simulink model "dPTPUDPNode1_tm"  (R2018b)
settings: Solver=FixedStepDiscrete  StartTime=0.0  StopTime=inf  FixedStep=0.01  RelTol=1e-3  EnableMultiTasking=on
undefined symbols (not defined in the file): ipaddr, PTP
libraries: xpcutilitieslib x6, xpcrtudplib x6, ptplib x3
settings Model: SimulationMode=external  Creator=The MathWorks, Inc.  LastModifiedBy=MAE-NCSUCORE
settings SolverCC: ConcurrentTasks=on  AutoInsertRateTranBlk=on  DecoupledContinuousIntegration=on  MinimalZcImpactIntegration=on
settings DataIOCC: SaveFormat=StructureWithTime
settings OptimizationCC: BlockReduction=off  OptimizeBlockIOStorage=off  BufferReuse=off  GlobalBufferReuse=off  ExpressionFolding=off  LocalBlockOutputs=off  OptimizeDataStoreBuffers=off  BusAssignmentInplaceUpdate=off
settings DebuggingCC: LibraryContextMissingDiagnostic=none
settings HardwareCC: ProdBitPerPointer=32  ProdBitPerSizeT=32  ProdBitPerPtrDiffT=32  ProdLargestAtomicFloat=None  ProdWordSize=32  ProdLongLongMode=on  ProdHWDeviceType=Generic->32-bit x86 compatible
settings SFSimCC: SimUseLocalCustomCode=off
settings RTWCC: SystemTargetFile=slrt.tlc  TemplateMakefile=slrt_default_tmf  Description=Simulink Real-Time  RTWVerbose=off  RTWUseLocalCustomCode=off  CodeExecutionProfiling=on  RTWCompilerOptimization=on
settings SimulinkRealTimeCC: SupportVariableSizeSignals=on  PreserveStateflowLocalDataDimensions=off  RL32LogTETModifier=off  RL32ObjectName=tg1  xPCisDefaultEnv=off  xPCTargetPCEnvName=Machine2  xPCConcurrentTasks=on

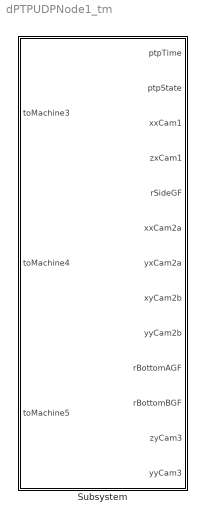
== system dPTPUDPNode1_tm ==
  Subsystem : Subsystem  TreatAsAtomicUnit=on  mask{sample_time=0.01, announce_interval=1, sync_interval=0.05}
      mask prompts: sample_time "Sample time (-1 for inherited)"; announce_interval "Announce interval (second):"; sync_interval "Sync interval (second):"
      mask TypeOptions sample_time: IEEE 1588 Read State/sample_time | IEEE 1588 Read Time/sample_time | IEEE 1588 Real-Time UDP/sample_time | UDP Receive Machine 3/sampleTime | UDP Receive Machine 4/sampleTime | UDP Receive Machine 5/sampleTime | UDP Send Machine 3/sampleTime | UDP Send Machine 4/sampleTime | UDP Send Machine 5/sampleTime
      mask TypeOptions announce_interval: IEEE 1588 Real-Time UDP/announce_interval
      mask TypeOptions sync_interval: IEEE 1588 Real-Time UDP/sync_interval

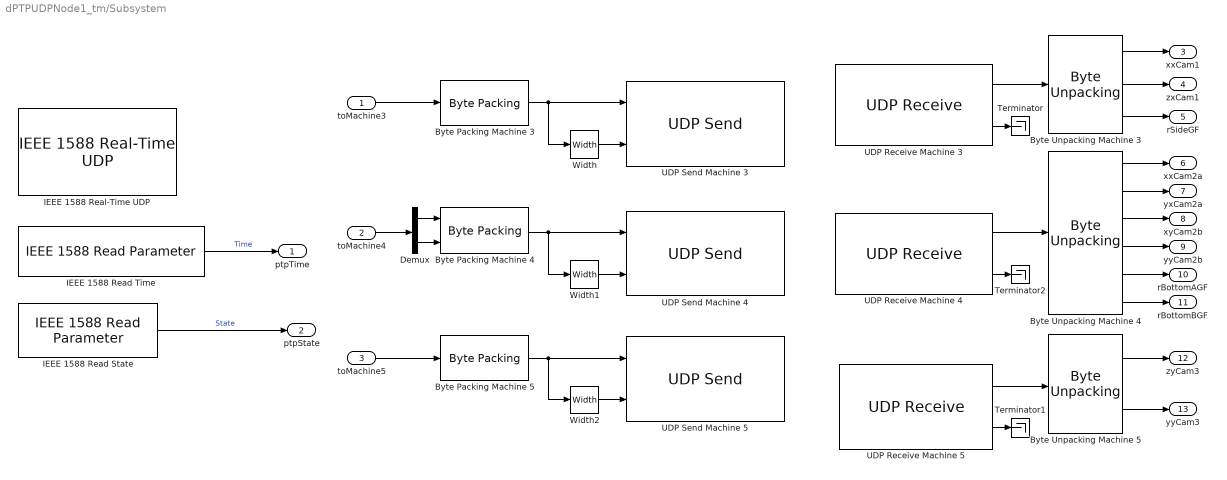
== system dPTPUDPNode1_tm/Subsystem ==
  toMachine3 : Inport
  toMachine4 : Inport  Port=2
  toMachine5 : Inport  Port=3
  Byte Packing Machine 3 : xpcutilitieslib/Byte Packing   MaskPackedDataType=uint8  MaskUnpackedDataTypes={['uint8']}  MaskAlignment=1
  Byte Packing Machine 4 : xpcutilitieslib/Byte Packing   MaskPackedDataType=uint8  MaskUnpackedDataTypes={['uint8'],['uint8']}  MaskAlignment=1
  Byte Packing Machine 5 : xpcutilitieslib/Byte Packing   MaskPackedDataType=uint8  MaskUnpackedDataTypes={['uint8']}  MaskAlignment=1
  "Byte Unpacking Machine 3 " : xpcutilitieslib/Byte Unpacking   MaskUnpackedDataTypes={'double','double',['uint8']}  MaskUnpackedDataSizes={[1],[1],[3]}  MaskAlignment=1
      settings: SourceProductName=Simulink Real-Time  SourceProductBaseCode=XP
  Byte Unpacking Machine 4 : xpcutilitieslib/Byte Unpacking   MaskUnpackedDataTypes={'double','double','double','double',['uint8'],['uint8']}  MaskUnpackedDataSizes={[1],[1],[1],[1],[3],[3]}  MaskAlignment=1
      settings: SourceProductName=Simulink Real-Time  SourceProductBaseCode=XP
  Byte Unpacking Machine 5 : xpcutilitieslib/Byte Unpacking   MaskUnpackedDataTypes={'double','double'}  MaskUnpackedDataSizes={[1],[1]}  MaskAlignment=1
      settings: SourceProductName=Simulink Real-Time  SourceProductBaseCode=XP
  Demux : Demux  Outputs=2
  IEEE 1588 Read State : ptplib/IEEE 1588 Read Parameter  Priority=1  ID=1  param=Protocol state  sample_time=sample_time  enable_read_precision=off
      settings: SourceProductName=Simulink Real-Time  SourceProductBaseCode=XP
  IEEE 1588 Read Time : ptplib/IEEE 1588 Read Parameter  Priority=1  ID=1  param=PTP time (time-of-day)  sample_time=sample_time  enable_read_precision=off
      settings: SourceProductName=Simulink Real-Time  SourceProductBaseCode=XP
  IEEE 1588 Real-Time UDP : ptplib/IEEE 1588 Real-Time UDP  Priority=0  ID=1  PciBus=2  PciSlot=0  PciFunction=0  time_inc=4000000  sample_time=sample_time  IpSource=Specify  IpAddress=30.30.30.30  SubnetMask=255.255.255.0  Gateway=0.0.0.0  Receive1=0.0.0.0  dest_ip_select=Specify  custom_dest_ip_addr=255.255.255.255  MulticastList=[ipaddr('224.0.1.129'), ipaddr('224.0.0.107')]  Multicast={macaddr('01:00:5E:00:01:81'), macaddr('01:00:5E:00:00:6B')}  time_source=Ethernet board  timescale=PTP (1970-01-01)  epoch=[1970 01 01 00]  delay_measure=Request-response  slave_only=off  enable_advanced_config=on  domain_num=0  utc_offset=35  priority1=1  clock_class=248  clock_accuracy=hex2dec('FE')  priority2=1  announce_interval=announce_interval  sync_interval=sync_interval  min_pdelay_req_interval=0.1  announce_receipt_timeout=3
      settings: SourceProductName=Simulink Real-Time  SourceProductBaseCode=XP
  Terminator : Terminator
  Terminator1 : Terminator
  Terminator2 : Terminator
  UDP Receive Machine 3 : xpcrtudplib/UDP Receive  ipAddressVal=30.30.30.30  localPort=8001  rcvWidth=8  rcvFmAny=off  fmAddress=30.30.30.1  rcvMulticast=off  multicastAddress={30.30.30.1, 30.30.30.2, 30.30.30.3}  maxUDPQueue=8  sampleTime=sample_time
      settings: SourceProductName=Simulink Real-Time
  UDP Receive Machine 4 : xpcrtudplib/UDP Receive  ipAddressVal=30.30.30.30  localPort=8002  rcvWidth=8  rcvFmAny=off  fmAddress=30.30.30.2  rcvMulticast=off  multicastAddress={30.30.30.1, 30.30.30.2, 30.30.30.3}  maxUDPQueue=8  sampleTime=sample_time
      settings: SourceProductName=Simulink Real-Time
  UDP Receive Machine 5 : xpcrtudplib/UDP Receive  ipAddressVal=30.30.30.30  localPort=8003  rcvWidth=8  rcvFmAny=off  fmAddress=30.30.30.3  rcvMulticast=off  multicastAddress={30.30.30.1, 30.30.30.2, 30.30.30.3}  maxUDPQueue=8  sampleTime=sample_time
      settings: SourceProductName=Simulink Real-Time
  UDP Send Machine 3 : xpcrtudplib/UDP Send  ipAddressVal=30.30.30.30  localPort=8001  toAddress=30.30.30.1  toPort=8000  sampleTime=sample_time
      settings: SourceProductName=Simulink Real-Time  SourceProductBaseCode=XP
  UDP Send Machine 4 : xpcrtudplib/UDP Send  ipAddressVal=30.30.30.30  localPort=8002  toAddress=30.30.30.2  toPort=8000  sampleTime=sample_time
      settings: SourceProductName=Simulink Real-Time  SourceProductBaseCode=XP
  UDP Send Machine 5 : xpcrtudplib/UDP Send  ipAddressVal=30.30.30.30  localPort=8003  toAddress=30.30.30.3  toPort=8000  sampleTime=sample_time
      settings: SourceProductName=Simulink Real-Time  SourceProductBaseCode=XP
  Width : Width
  Width1 : Width
  Width2 : Width
  ptpTime : Outport
  ptpState : Outport  Port=2
  xxCam1 : Outport  Port=3
  zxCam1 : Outport  Port=4
  rSideGF : Outport  Port=5
  xxCam2a : Outport  Port=6
  yxCam2a : Outport  Port=7
  xyCam2b : Outport  Port=8
  yyCam2b : Outport  Port=9
  rBottomAGF : Outport  Port=10
  rBottomBGF : Outport  Port=11
  zyCam3 : Outport  Port=12
  yyCam3 : Outport  Port=13
  wires:
  Byte Unpacking Machine 4/1 -> xxCam2a/1
  Byte Unpacking Machine 4/6 -> rBottomBGF/1
  Byte Unpacking Machine 4/3 -> xyCam2b/1
  UDP Receive Machine 5/1 -> Byte Unpacking Machine 5/1
  "Byte Unpacking Machine 3 "/3 -> rSideGF/1
  toMachine3/1 -> Byte Packing Machine 3/1
  IEEE 1588 Read State/1 -> ptpState/1  "State"
  "Byte Unpacking Machine 3 "/2 -> zxCam1/1
  toMachine5/1 -> Byte Packing Machine 5/1
  toMachine4/1 -> Demux/1
  Demux/2 -> Byte Packing Machine 4/2
  Byte Unpacking Machine 5/1 -> zyCam3/1
  UDP Receive Machine 4/2 -> Terminator2/1
  Width/1 -> UDP Send Machine 3/2
  "Byte Unpacking Machine 3 "/1 -> xxCam1/1
  UDP Receive Machine 5/2 -> Terminator1/1
  Byte Unpacking Machine 4/2 -> yxCam2a/1
  UDP Receive Machine 3/2 -> Terminator/1
  Byte Packing Machine 3/1 -> UDP Send Machine 3/1, Width/1
  Width2/1 -> UDP Send Machine 5/2
  Demux/1 -> Byte Packing Machine 4/1
  Byte Unpacking Machine 4/4 -> yyCam2b/1
  IEEE 1588 Read Time/1 -> ptpTime/1  "Time"
  Byte Packing Machine 4/1 -> UDP Send Machine 4/1, Width1/1
  UDP Receive Machine 4/1 -> Byte Unpacking Machine 4/1
  UDP Receive Machine 3/1 -> "Byte Unpacking Machine 3 "/1
  Byte Unpacking Machine 5/2 -> yyCam3/1
  Width1/1 -> UDP Send Machine 4/2
  Byte Unpacking Machine 4/5 -> rBottomAGF/1
  Byte Packing Machine 5/1 -> UDP Send Machine 5/1, Width2/1
